simulink model "my_model"  (Simulink 10.0)
settings: Solver=ode45  StartTime=0.0  StopTime=inf  RelTol=1e-3  EnableMultiTasking=on
settings Model: Creator=Q.Ahmed  LastModifiedBy=unknown
settings DataIOCC: LimitDataPoints=on  SignalLoggingSaveFormat=ModelDataLogs
settings OptimizationCC: InitFltsAndDblsToZero=on
settings DebuggingCC: SaveWithParameterizedLinksMsg=none  SignalResolutionControl=TryResolveAllWithWarning  SolverPrmCheckMsg=warning  FcnCallInpInsideContextMsg=warning
settings SFSimCC: SimUseLocalCustomCode=on  CustomCodeUndefinedFunction=FilterOut
settings RTWCC: RTWUseLocalCustomCode=on
settings GRTTargetCC: TargetFcnLib=ansi_tfl_tmw.mat

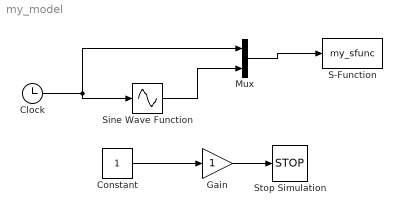
== system my_model ==
  Clock : Clock
  Constant : Constant
  Gain : Gain
  Mux : Mux  Inputs=2
  S-Function : S-Function  FunctionName=my_sfunc  SFunctionDeploymentMode=off  EnableBusSupport=off
  Sine Wave Function : Sin  TimeSource=Use external signal  SampleTime=0
  Stop Simulation : Stop
  wires:
  Clock/1 -> Sine Wave Function/1, Mux/1
  Sine Wave Function/1 -> Mux/2
  Gain/1 -> Stop Simulation/1
  Constant/1 -> Gain/1
  Mux/1 -> S-Function/1
